simulink model "regulateur_comparaion"  (R2019b)
settings: Solver=VariableStepAuto  StartTime=0.0  StopTime=2  RelTol=1e-3
settings Model: Creator=jeanz  LastModifiedBy=jeanz

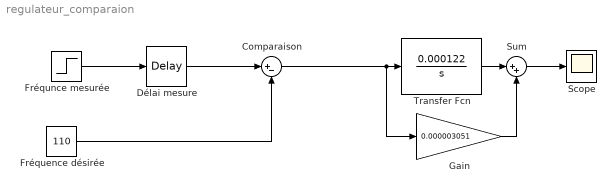
== system regulateur_comparaion ==
  Comparaison : Sum  Inputs=|+-
  Délai mesure : TransportDelay  DelayTime=0.27
  Fréquence désirée : Constant  Value=110
  Fréqunce mesurée : Step  SampleTime=0
  Gain : Gain  Gain=0.000003051
  Scope : Scope
  Sum : Sum  Inputs=|++
  Transfer Fcn : TransferFcn  Numerator=[0.000122]  Denominator=[1 0]
  wires:
  Transfer Fcn/1 -> Sum/1
  Gain/1 -> Sum/2
  Sum/1 -> Scope/1
  Comparaison/1 -> Gain/1, Transfer Fcn/1
  Délai mesure/1 -> Comparaison/1
  Fréquence désirée/1 -> Comparaison/2
  Fréqunce mesurée/1 -> Délai mesure/1
